simulink model "practice2"  (Simulink 7.9)
settings: Solver=ode45  StartTime=0.0  StopTime=60  RelTol=1e-3
settings Model: Creator=sony  LastModifiedBy=sony

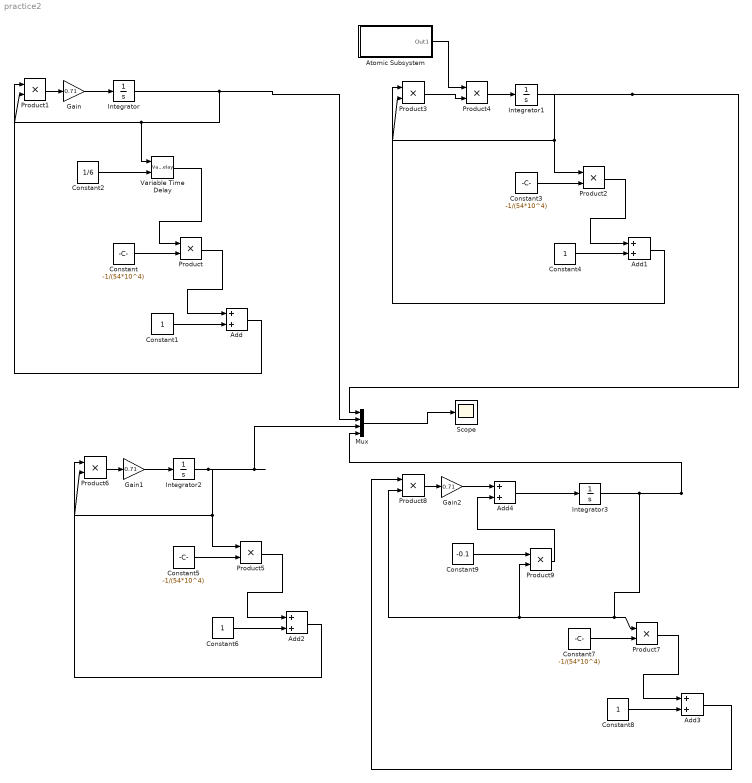
== system practice2 ==
  Add{,1..4} (5 alike) : Sum
  Atomic Subsystem : Subsystem  TreatAsAtomicUnit=on
  Constant{,3,5,7} (4 alike) : Constant  Value=-1/(54*10^4)
  Constant{1,4,6,8} (4 alike) : Constant
  Constant2 : Constant  Value=1/6
  Constant9 : Constant  Value=-0.1
  Gain : Gain  Gain=0.71
  Gain1 : Gain  Gain=0.71
  Gain2 : Gain  Gain=0.71
  Integrator{,1..3} (4 alike) : Integrator  InitialCondition=(1/4)*54*10^4
  Mux : Mux
  Product{,1..9} (10 alike) : Product  RndMeth=Zero
  Scope : Scope
  Variable Time Delay : VariableTransportDelay  MaximumDelay=10
  wires:
  Constant/1 -> Product/2
  Product/1 -> Add/1
  Constant1/1 -> Add/2
  Add/1 -> Product1/1
  Product1/1 -> Gain/1
  Gain/1 -> Integrator/1
  Constant2/1 -> Variable Time Delay/2
  Variable Time Delay/1 -> Product/1
  Constant3/1 -> Product2/2
  Product2/1 -> Add1/1
  Constant4/1 -> Add1/2
  Add1/1 -> Product3/1
  Integrator1/1 -> Product2/1, Product3/2, Mux/1
  Product4/1 -> Integrator1/1
  Product3/1 -> Product4/2
  Atomic Subsystem/1(Out1) -> Product4/1
  Integrator/1 -> Product1/2, Variable Time Delay/1, Mux/2
  Constant7/1 -> Product7/2
  Product7/1 -> Add3/1
  Constant8/1 -> Add3/2
  Add3/1 -> Product8/1
  Product8/1 -> Gain2/1
  Constant9/1 -> Product9/1
  Product9/1 -> Add4/2
  Gain2/1 -> Add4/1
  Add4/1 -> Integrator3/1
  Integrator3/1 -> Product7/1, Product8/2, Product9/2, Mux/4
  Constant5/1 -> Product5/2
  Product5/1 -> Add2/1
  Constant6/1 -> Add2/2
  Add2/1 -> Product6/1
  Integrator2/1 -> Product5/1, Product6/2, Mux/3
  Product6/1 -> Gain1/1
  Gain1/1 -> Integrator2/1
  Mux/1 -> Scope/1

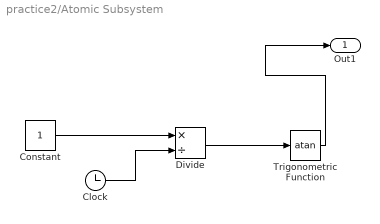
== system practice2/Atomic Subsystem ==
  Clock : Clock
  Constant : Constant
  Divide : Product  Inputs=*/
  Trigonometric Function : Trigonometry  Operator=atan
  Out1 : Outport
  wires:
  Constant/1 -> Divide/1
  Clock/1 -> Divide/2
  Divide/1 -> Trigonometric Function/1
  Trigonometric Function/1 -> Out1/1
